simulink model "example2_0511_pendulum"  (R2023b)
settings: Solver=VariableStepAuto  StartTime=0.0  StopTime=tFinal  MaxStep=maxStepSize  RelTol=1e-3
values from neighbouring files (symbols this model uses):
  c = 0.2    [parametersfromMatlab_0611.m]
  g = 10    [parametersfromMatlab_0611.m]
  l = 1    [parametersfromMatlab_0611.m]
  m = 1    [parametersfromMatlab_0611.m]
settings Model: Creator=martinhaugen  LastModifiedBy=martinhaugen

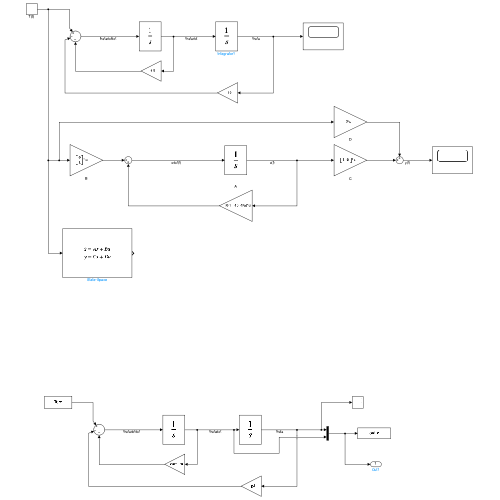
[thumbnail: Simulink's stored preview of the top-level diagram]
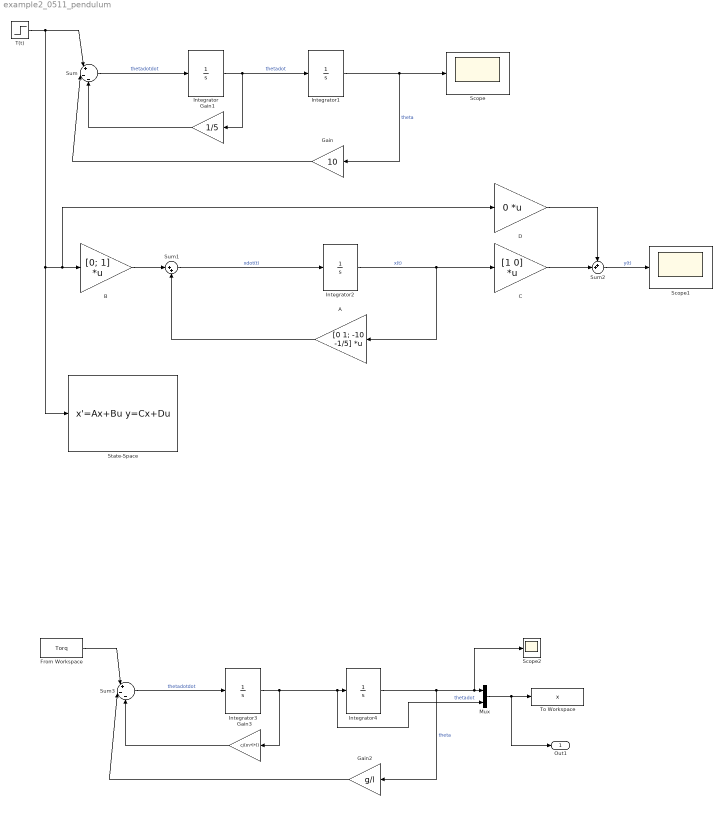
== system example2_0511_pendulum ==
  A : Gain  Gain=[0 1; -10 -1/5]  Multiplication=Matrix(K*u)
  B : Gain  Gain=[0; 1]  Multiplication=Matrix(K*u)
  C : Gain  Gain=[1 0]  Multiplication=Matrix(K*u)
  D : Gain  Gain=0  Multiplication=Matrix(K*u)
  From Workspace : FromWorkspace  VariableName=Torq
  Gain : Gain  Gain=10
  Gain1 : Gain  Gain=1/5
  Gain2 : Gain  Gain=g/l
  Gain3 : Gain  Gain=c/(m*l*l)
  Integrator{,1..4} (5 alike) : Integrator
  Mux : Mux  Inputs=2
  Scope : Scope
  Scope1 : Scope
  Scope2 : Scope
  State-Space : StateSpace  A=[0 1; -10 -1/5]  B=[0; 1]  C=[1 0]  D=0  InitialCondition=0
  Sum : Sum  Inputs=|+|-|-
  Sum1 : Sum  Inputs=|++
  Sum2 : Sum  Inputs=++|
  Sum3 : Sum  Inputs=|+|-|-
  T(t) : Step  SampleTime=0
  To Workspace : ToWorkspace  VariableName=x  SaveFormat=Timeseries  SampleTime=-1
  Out1 : Outport
  wires:
  Integrator/1 -> Gain1/1, Integrator1/1  "thetadot"
  Sum/1 -> Integrator/1  "thetadotdot"
  Integrator1/1 -> Scope/1, Gain/1  "theta"
  T(t)/1 -> Sum/1, B/1, D/1, State-Space/1
  Gain/1 -> Sum/2
  Gain1/1 -> Sum/3
  Sum1/1 -> Integrator2/1  "xdot(t)"
  Integrator2/1 -> C/1, A/1  "x(t)"
  A/1 -> Sum1/2
  B/1 -> Sum1/1
  C/1 -> Sum2/2
  D/1 -> Sum2/1
  Sum2/1 -> Scope1/1  "y(t)"
  Integrator3/1 -> Gain3/1, Mux/2, Integrator4/1  "thetadot"
  From Workspace/1 -> Sum3/1
  Gain2/1 -> Sum3/2
  Sum3/1 -> Integrator3/1  "thetadotdot"
  Integrator4/1 -> Scope2/1, Mux/1, Gain2/1  "theta"
  Gain3/1 -> Sum3/3
  Mux/1 -> To Workspace/1, Out1/1
